simulink model "counterupdown"  (R2021b)
settings: Solver=VariableStepAuto  StartTime=0.0  StopTime=10.0  RelTol=1e-3
settings Model: Creator=midol  LastModifiedBy=midol

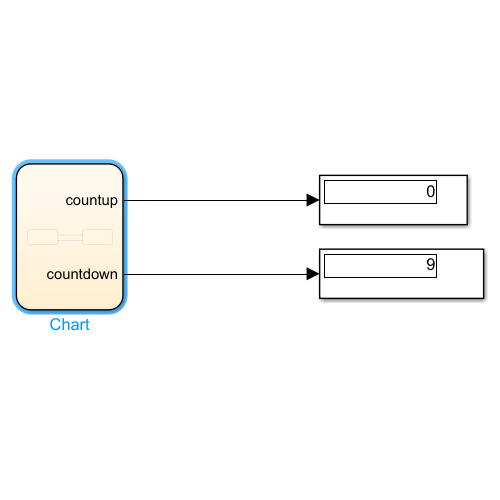
[thumbnail: Simulink's stored preview of the top-level diagram]
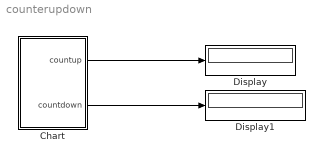
== system counterupdown ==
  Chart : Stateflow chart  TreatAsAtomicUnit=on
  Display : Display
  Display1 : Display
  wires:
  Chart/1(countup) -> Display/1
  Chart/2(countdown) -> Display1/1

== stateflow chart counterupdown/Chart ==
  state increment [parallel]
    en:
    countup = 0;
    du:
    countup = countup+1;
    ex:
    countup = 0;
    settings: executionOrder=1
  state decrement [parallel]
    en:
    countdown = 10;
    du:
    countdown = countdown-1;
    ex:
    countdown = 10;
    settings: executionOrder=2
  increment -> decrement : [countup == 10]
  decrement -> increment : [countdown == 0]
  data: countup output; countdown output
